simulink subsystem "PvtSubSys_VSM_SCM"  (R2020b)
settings: Solver=VariableStepAuto  StartTime=0.0  StopTime=10.0  RelTol=1e-3
undefined symbols (not defined in the file): P_Global_VehicleWidthMin_m, P_VSM_LDW_State_Param_LaneTime, P_VSM_LDW_State_Param_Speed, P_VSM_LKA_State_Param_Offset, P_VSM_LSMC_SampleTime
libraries: simulink x45
(part 3 of 3)

== matlab function PvtSubSys_VSM_SCM/LKA_LDW_SignalProcess/DTLC ==
  data: LDWLKA_PreT input; VehicleSpd_ms input; Kap input; VehicleWidth_m input; FLWhelDy output single; FRWhelDy output single; LA0 input; LA1 input; LA2 input; LA3 input; Lvalid input; RA0 input; RA1 input; RA2 input; RA3 input; Rvalid input; preFLWhelDy output single; preFRWhelDy output single
function [FLWhelDy,FRWhelDy,preFLWhelDy,preFRWhelDy]  = DTLC(LDWLKA_PreT,VehicleSpd_ms,Kap,VehicleWidth_m,LA0,LA1,LA2,LA3,Lvalid,RA0,RA1,RA2,RA3,Rvalid)
% 
%
    predx=LDWLKA_PreT*VehicleSpd_ms;
    halfVechileWidth=single(VehicleWidth_m/2);
 if Kap<0.0001
     EgoDy=single(0);
 else
     EgoDy= 1/Kap-predx/(tan(asin(predx*Kap)));
 end

    
    

    if Lvalid>0
        preFLWhelDy=LA0+LA1*predx+LA2*predx^2+LA3*predx^3 - EgoDy - halfVechileWidth;
        FLWhelDy=(LA0-halfVechileWidth)/single(sqrt(LA1*LA1+1));
    else
        preFLWhelDy=single(0);
        FLWhelDy=single(0);
    end
    if Rvalid>0
        preFRWhelDy=-(RA0+RA1*predx+RA2*predx^2+RA3*predx^3 - EgoDy + halfVechileWidth);
        FRWhelDy=-(RA0+halfVechileWidth)/single(sqrt(RA1*RA1+1));
    else
        preFRWhelDy=single(0);
        FRWhelDy=single(0);
    end
